simulink model "simulacija"  (R2015b)
settings: Solver=ode4  StartTime=0.0  StopTime=0.2  FixedStep=0.001  RelTol=1e-3
values from neighbouring files (symbols this model uses):
  delta_z = L/(N-1)    (= 7.5)    [assignment.m]
  dpdz = 80    [assignment.m]
  Q0 = 16.7    [assignment.m]
  ro = 15    [assignment.m]
  s0 = 1.2    [assignment.m]
  v = 0.035    [assignment.m]
settings Model: Creator=eBrand  LastModifiedBy=eBrand

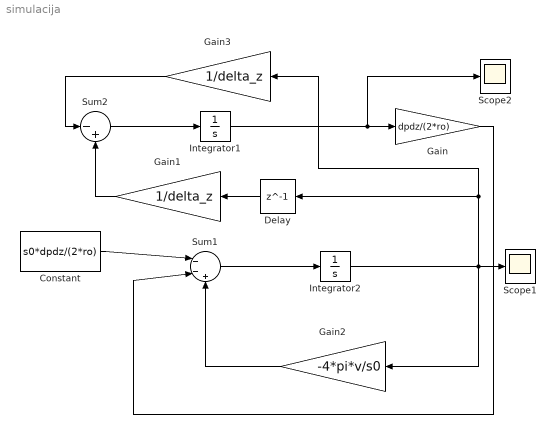
== system simulacija ==
  Constant : Constant  Value=s0*dpdz/(2*ro)
  Delay : Delay  DelayLength=1  InitialCondition=Q0
  Gain : Gain  Gain=dpdz/(2*ro)
  Gain1 : Gain  Gain=1/delta_z
  Gain2 : Gain  Gain=-4*pi*v/s0
  Gain3 : Gain  Gain=1/delta_z
  Integrator1 : Integrator  InitialCondition=s0
  Integrator2 : Integrator  InitialCondition=Q0
  Scope1 : Scope
  Scope2 : Scope
  Sum1 : Sum  Inputs=|--+
  Sum2 : Sum  Inputs=|-+
  wires:
  Integrator2/1 -> Gain3/1, Delay/1, Gain2/1, Scope1/1
  Sum1/1 -> Integrator2/1
  Gain2/1 -> Sum1/3
  Constant/1 -> Sum1/1
  Gain/1 -> Sum1/2
  Sum2/1 -> Integrator1/1
  Delay/1 -> Gain1/1
  Gain1/1 -> Sum2/2
  Integrator1/1 -> Scope2/1, Gain/1
  Gain3/1 -> Sum2/1
